simulink model "power_PSTdeltahex"  (Simulink 6.0)
settings: Solver=ode23tb  StartTime=0.0  StopTime=50  MaxStep=1/60  RelTol=1e-4  AbsTol=1e-3
undefined symbols (not defined in the file or in its folder): I21_init_imag, I21_init_real
libraries: powerlib x117, powerlib_extras x19, simulink_extras x1
(part 3 of 3)

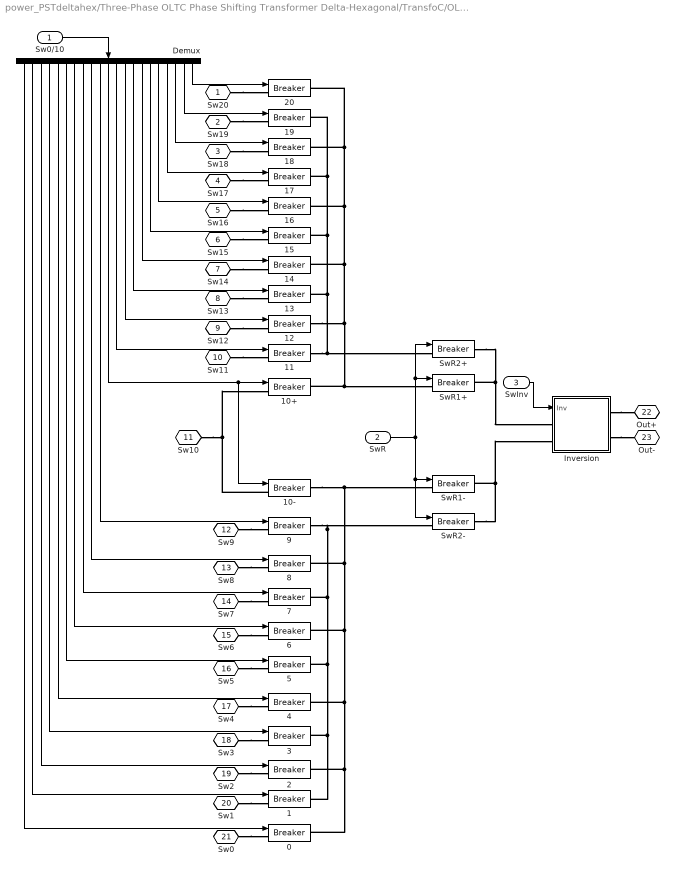
== system power_PSTdeltahex/Three-Phase OLTC Phase Shifting Transformer Delta-Hexagonal/TransfoC/OLTC ==
  Sw0/10 : Inport  Port=1  LatchInput=off
  SwR : Inport  Port=2  LatchInput=off
  SwInv : Inport  Port=3  LatchInput=off
  "0  " : powerlib/Elements/Breaker  BreakerResistance=Ron  InitialState=InitialStates(1)  SnubberResistance=Rsnub  SnubberCapacitance=inf  SwitchingTimes="[ 1/60  5/60 ]"  External=on  Measurements=None
  "1  " : powerlib/Elements/Breaker  BreakerResistance=Ron  InitialState=InitialStates(2)  SnubberResistance=Rsnub  SnubberCapacitance=inf  SwitchingTimes="[ 1/60  5/60 ]"  External=on  Measurements=None
  "10+  " : powerlib/Elements/Breaker  BreakerResistance=Ron  InitialState=InitialStates(11)  SnubberResistance=1e6  SnubberCapacitance=Rsnub  SwitchingTimes="[ 1/60  5/60 ]"  External=on  Measurements=None
  10- : powerlib/Elements/Breaker  BreakerResistance=Ron  InitialState=InitialStates(11)  SnubberResistance=Rsnub  SnubberCapacitance=inf  SwitchingTimes="[ 1/60  5/60 ]"  External=on  Measurements=None
  11 : powerlib/Elements/Breaker  BreakerResistance=Ron  InitialState=InitialStates(12)  SnubberResistance=Rsnub  SnubberCapacitance=inf  SwitchingTimes="[ 1/60  5/60 ]"  External=on  Measurements=None
  12 : powerlib/Elements/Breaker  BreakerResistance=Ron  InitialState=InitialStates(13)  SnubberResistance=Rsnub  SnubberCapacitance=inf  SwitchingTimes="[ 1/60  5/60 ]"  External=on  Measurements=None
  13 : powerlib/Elements/Breaker  BreakerResistance=Ron  InitialState=InitialStates(14)  SnubberResistance=Rsnub  SnubberCapacitance=inf  SwitchingTimes="[ 1/60  5/60 ]"  External=on  Measurements=None
  14 : powerlib/Elements/Breaker  BreakerResistance=Ron  InitialState=InitialStates(15)  SnubberResistance=Rsnub  SnubberCapacitance=inf  SwitchingTimes="[ 1/60  5/60 ]"  External=on  Measurements=None
  15 : powerlib/Elements/Breaker  BreakerResistance=Ron  InitialState=InitialStates(16)  SnubberResistance=Rsnub  SnubberCapacitance=inf  SwitchingTimes="[ 1/60  5/60 ]"  External=on  Measurements=None
  "16  " : powerlib/Elements/Breaker  BreakerResistance=Ron  InitialState=InitialStates(17)  SnubberResistance=Rsnub  SnubberCapacitance=inf  SwitchingTimes="[ 1/60  5/60 ]"  External=on  Measurements=None
  17 : powerlib/Elements/Breaker  BreakerResistance=Ron  InitialState=InitialStates(18)  SnubberResistance=Rsnub  SnubberCapacitance=inf  SwitchingTimes="[ 1/60  5/60 ]"  External=on  Measurements=None
  18 : powerlib/Elements/Breaker  BreakerResistance=Ron  InitialState=InitialStates(19)  SnubberResistance=Rsnub  SnubberCapacitance=inf  SwitchingTimes="[ 1/60  5/60 ]"  External=on  Measurements=None
  19 : powerlib/Elements/Breaker  BreakerResistance=Ron  InitialState=InitialStates(20)  SnubberResistance=Rsnub  SnubberCapacitance=inf  SwitchingTimes="[ 1/60  5/60 ]"  External=on  Measurements=None
  "2    " : powerlib/Elements/Breaker  BreakerResistance=Ron  InitialState=InitialStates(3)  SnubberResistance=Rsnub  SnubberCapacitance=inf  SwitchingTimes="[ 1/60  5/60 ]"  External=on  Measurements=None
  20 : powerlib/Elements/Breaker  BreakerResistance=Ron  InitialState=InitialStates(21)  SnubberResistance=Rsnub  SnubberCapacitance=inf  SwitchingTimes="[ 1/60  5/60 ]"  External=on  Measurements=None
  "3  " : powerlib/Elements/Breaker  BreakerResistance=Ron  InitialState=InitialStates(4)  SnubberResistance=Rsnub  SnubberCapacitance=inf  SwitchingTimes="[ 1/60  5/60 ]"  External=on  Measurements=None
  "4  " : powerlib/Elements/Breaker  BreakerResistance=Ron  InitialState=InitialStates(5)  SnubberResistance=Rsnub  SnubberCapacitance=inf  SwitchingTimes="[ 1/60  5/60 ]"  External=on  Measurements=None
  5 : powerlib/Elements/Breaker  BreakerResistance=Ron  InitialState=InitialStates(6)  SnubberResistance=Rsnub  SnubberCapacitance=inf  SwitchingTimes="[ 1/60  5/60 ]"  External=on  Measurements=None
  6 : powerlib/Elements/Breaker  BreakerResistance=Ron  InitialState=InitialStates(7)  SnubberResistance=Rsnub  SnubberCapacitance=inf  SwitchingTimes="[ 1/60  5/60 ]"  External=on  Measurements=None
  7 : powerlib/Elements/Breaker  BreakerResistance=Ron  InitialState=InitialStates(8)  SnubberResistance=Rsnub  SnubberCapacitance=inf  SwitchingTimes="[ 1/60  5/60 ]"  External=on  Measurements=None
  8 : powerlib/Elements/Breaker  BreakerResistance=Ron  InitialState=InitialStates(9)  SnubberResistance=Rsnub  SnubberCapacitance=inf  SwitchingTimes="[ 1/60  5/60 ]"  External=on  Measurements=None
  9 : powerlib/Elements/Breaker  BreakerResistance=Ron  InitialState=InitialStates(10)  SnubberResistance=Rsnub  SnubberCapacitance=inf  SwitchingTimes="[ 1/60  5/60 ]"  External=on  Measurements=None
  Demux : Demux  Orientation=down  Outputs=21
  Inversion : Subsystem
  SwR1+ : powerlib/Elements/Breaker  BreakerResistance=Ron  InitialState=1  SnubberResistance=R  SnubberCapacitance=inf  SwitchingTimes="[ 1/60  5/60 ]"  External=on  Measurements=None
  SwR1- : powerlib/Elements/Breaker  BreakerResistance=Ron  InitialState=1  SnubberResistance=R  SnubberCapacitance=inf  SwitchingTimes="[ 1/60  5/60 ]"  External=on  Measurements=None
  SwR2+ : powerlib/Elements/Breaker  BreakerResistance=Ron  InitialState=1  SnubberResistance=R  SnubberCapacitance=inf  SwitchingTimes="[ 1/60  5/60 ]"  External=on  Measurements=None
  SwR2- : powerlib/Elements/Breaker  BreakerResistance=Ron  InitialState=1  SnubberResistance=R  SnubberCapacitance=inf  SwitchingTimes="[ 1/60  5/60 ]"  External=on  Measurements=None
  Sw20 : PMIOPort  Port=1  Side=Left
  Sw19 : PMIOPort  Port=2  Side=Left
  Sw18 : PMIOPort  Port=3  Side=Left
  Sw17 : PMIOPort  Port=4  Side=Left
  Sw16 : PMIOPort  Port=5  Side=Left
  Sw15 : PMIOPort  Port=6  Side=Left
  Sw14 : PMIOPort  Port=7  Side=Left
  Sw13 : PMIOPort  Port=8  Side=Left
  Sw12 : PMIOPort  Port=9  Side=Left
  Sw11 : PMIOPort  Port=10  Side=Left
  Sw10 : PMIOPort  Port=11  Side=Left
  "Sw9 " : PMIOPort  Port=12  Side=Left
  Sw8 : PMIOPort  Port=13  Side=Left
  Sw7 : PMIOPort  Port=14  Side=Left
  Sw6 : PMIOPort  Port=15  Side=Left
  Sw5 : PMIOPort  Port=16  Side=Left
  Sw4 : PMIOPort  Port=17  Side=Left
  Sw3 : PMIOPort  Port=18  Side=Left
  "Sw2 " : PMIOPort  Port=19  Side=Left
  Sw1 : PMIOPort  Port=20  Side=Left
  Sw0 : PMIOPort  Port=21  Side=Left
  Out+ : PMIOPort  Orientation=left  Port=22  Side=Right
  Out- : PMIOPort  Orientation=left  Port=23  Side=Right
  wires:
  Sw0/10/1 -> Demux/1
  Demux/1 -> "0  "/1
  Demux/2 -> "1  "/1
  Demux/3 -> "2    "/1
  Demux/4 -> "3  "/1
  Demux/5 -> "4  "/1
  SwInv/1 -> Inversion/1(Inv)
  Demux/21 -> 20/1
  Demux/20 -> 19/1
  Demux/19 -> 18/1
  Demux/18 -> 17/1
  Demux/17 -> "16  "/1
  Demux/16 -> 15/1
  Demux/15 -> 14/1
  Demux/14 -> 13/1
  Demux/13 -> 12/1
  Demux/12 -> 11/1
  Demux/11 -> "10+  "/1, 10-/1
  Demux/10 -> 9/1
  Demux/9 -> 8/1
  Demux/8 -> 7/1
  Demux/7 -> 6/1
  Demux/6 -> 5/1
  SwR/1 -> SwR2+/1, SwR1+/1, SwR1-/1, SwR2-/1
  connections:
  Sw20/RConn1 -- 20/LConn1
  Sw19/RConn1 -- 19/LConn1
  Sw18/RConn1 -- 18/LConn1
  Sw17/RConn1 -- 17/LConn1
  Sw16/RConn1 -- "16  "/LConn1
  Sw4/RConn1 -- "4  "/LConn1
  Sw3/RConn1 -- "3  "/LConn1
  "Sw2 "/RConn1 -- "2    "/LConn1
  Sw1/RConn1 -- "1  "/LConn1
  Sw0/RConn1 -- "0  "/LConn1
  Inversion/RConn1 -- Out+/RConn1
  Inversion/RConn2 -- Out-/RConn1
  Sw5/RConn1 -- 5/LConn1
  Sw6/RConn1 -- 6/LConn1
  Sw7/RConn1 -- 7/LConn1
  Sw8/RConn1 -- 8/LConn1
  "Sw9 "/RConn1 -- 9/LConn1
  Sw15/RConn1 -- 15/LConn1
  Sw14/RConn1 -- 14/LConn1
  Sw13/RConn1 -- 13/LConn1
  Sw12/RConn1 -- 12/LConn1
  Sw11/RConn1 -- 11/LConn1
  SwR2-/RConn1 -- SwR1-/RConn1 -- Inversion/LConn2
  10-/RConn1 -- 8/RConn1 -- 6/RConn1 -- "4  "/RConn1 -- "2    "/RConn1 -- "0  "/RConn1 -- SwR1-/LConn1
  9/RConn1 -- 7/RConn1 -- 5/RConn1 -- "3  "/RConn1 -- "1  "/RConn1 -- SwR2-/LConn1
  12/RConn1 -- 14/RConn1 -- "16  "/RConn1 -- 18/RConn1 -- 20/RConn1 -- "10+  "/RConn1 -- SwR1+/LConn1
  11/RConn1 -- 13/RConn1 -- 15/RConn1 -- 17/RConn1 -- 19/RConn1 -- SwR2+/LConn1
  10-/LConn1 -- "10+  "/LConn1 -- Sw10/RConn1
  SwR2+/RConn1 -- SwR1+/RConn1 -- Inversion/LConn1

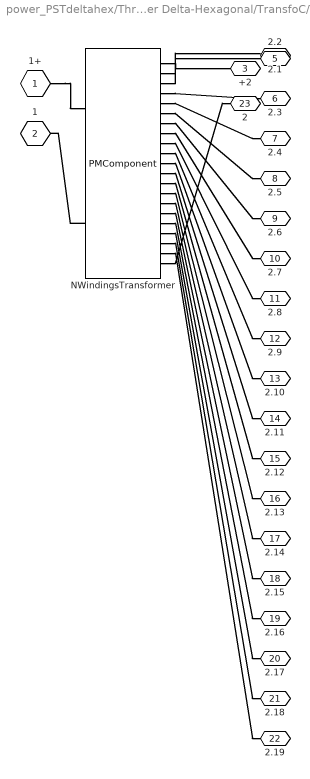
== system power_PSTdeltahex/Three-Phase OLTC Phase Shifting Transformer Delta-Hexagonal/TransfoC/Transformer ==
  NWindingsTransformer : PMComponent  PhysicalDomain=powersysdomain  LeftPortType=p1  RightPortType=p1  LConnTagsString=1|2  RConnTagsString=1|2|3|4|5|6|7|8|9|10|11|12|13|14|15|16|17|18|19|20|21
      mask Type: InnerPowersysBlock
  1+ : PMIOPort  Port=1  Side=Left
  1 : PMIOPort  Port=2  Side=Left
  +2 : PMIOPort  Orientation=left  Port=3  Side=Right
  2.1 : PMIOPort  Orientation=left  Port=4  Side=Right
  2.2 : PMIOPort  Orientation=left  Port=5  Side=Right
  2.3 : PMIOPort  Orientation=left  Port=6  Side=Right
  2.4 : PMIOPort  Orientation=left  Port=7  Side=Right
  2.5 : PMIOPort  Orientation=left  Port=8  Side=Right
  2.6 : PMIOPort  Orientation=left  Port=9  Side=Right
  2.7 : PMIOPort  Orientation=left  Port=10  Side=Right
  2.8 : PMIOPort  Orientation=left  Port=11  Side=Right
  2.9 : PMIOPort  Orientation=left  Port=12  Side=Right
  2.10 : PMIOPort  Orientation=left  Port=13  Side=Right
  2.11 : PMIOPort  Orientation=left  Port=14  Side=Right
  2.12 : PMIOPort  Orientation=left  Port=15  Side=Right
  2.13 : PMIOPort  Orientation=left  Port=16  Side=Right
  2.14 : PMIOPort  Orientation=left  Port=17  Side=Right
  2.15 : PMIOPort  Orientation=left  Port=18  Side=Right
  2.16 : PMIOPort  Orientation=left  Port=19  Side=Right
  2.17 : PMIOPort  Orientation=left  Port=20  Side=Right
  2.18 : PMIOPort  Orientation=left  Port=21  Side=Right
  2.19 : PMIOPort  Orientation=left  Port=22  Side=Right
  2 : PMIOPort  Orientation=left  Port=23  Side=Right
  connections:
  NWindingsTransformer/RConn1 -- +2/RConn1
  1+/RConn1 -- NWindingsTransformer/LConn1
  NWindingsTransformer/LConn2 -- 1/RConn1
  NWindingsTransformer/RConn2 -- 2.1/RConn1
  NWindingsTransformer/RConn3 -- 2.2/RConn1
  NWindingsTransformer/RConn4 -- 2.3/RConn1
  NWindingsTransformer/RConn5 -- 2.4/RConn1
  NWindingsTransformer/RConn6 -- 2.5/RConn1
  NWindingsTransformer/RConn7 -- 2.6/RConn1
  NWindingsTransformer/RConn8 -- 2.7/RConn1
  NWindingsTransformer/RConn9 -- 2.8/RConn1
  NWindingsTransformer/RConn10 -- 2.9/RConn1
  NWindingsTransformer/RConn21 -- 2/RConn1
  NWindingsTransformer/RConn11 -- 2.10/RConn1
  NWindingsTransformer/RConn12 -- 2.11/RConn1
  NWindingsTransformer/RConn13 -- 2.12/RConn1
  NWindingsTransformer/RConn14 -- 2.13/RConn1
  NWindingsTransformer/RConn15 -- 2.14/RConn1
  NWindingsTransformer/RConn16 -- 2.15/RConn1
  NWindingsTransformer/RConn17 -- 2.16/RConn1
  NWindingsTransformer/RConn18 -- 2.17/RConn1
  NWindingsTransformer/RConn19 -- 2.18/RConn1
  NWindingsTransformer/RConn20 -- 2.19/RConn1

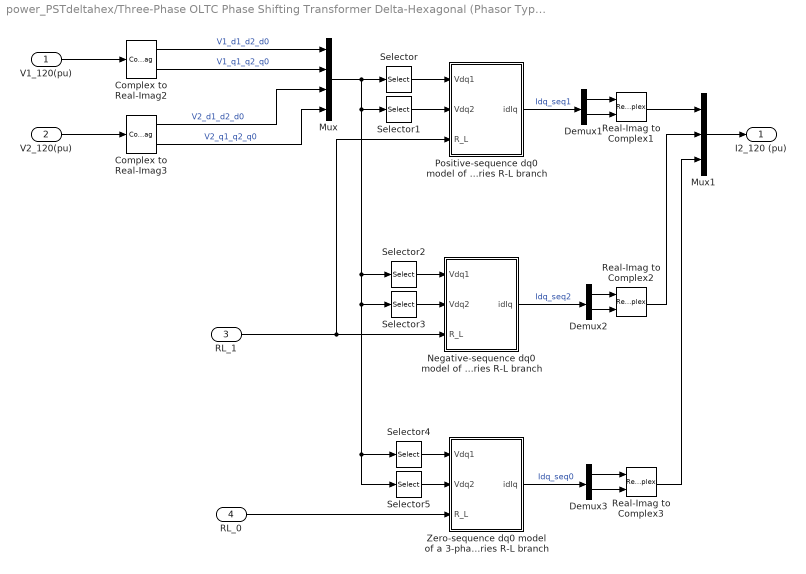
== system power_PSTdeltahex/Three-Phase OLTC Phase Shifting Transformer Delta-Hexagonal (Phasor Type)/ Currents/dq0 model of 3-ph RL branch ==
  V1_120(pu) : Inport  Port=1  LatchInput=off
  V2_120(pu) : Inport  Port=2  LatchInput=off
  RL_1 : Inport  Port=3  LatchInput=off
  RL_0 : Inport  Port=4  LatchInput=off
  Complex to Real-Imag2 : ComplexToRealImag
  Complex to Real-Imag3 : ComplexToRealImag
  Demux1 : Demux  Outputs=2
  Demux2 : Demux  Outputs=2
  Demux3 : Demux  Outputs=2
  Mux : Mux
  Mux1 : Mux  Inputs=3
  Negative-sequence dq0 model of a 3-phase series R-L branch : Subsystem
  Positive-sequence dq0 model of a 3-phase series R-L branch : Subsystem
  Real-Imag to Complex1 : RealImagToComplex
  Real-Imag to Complex2 : RealImagToComplex
  Real-Imag to Complex3 : RealImagToComplex
  Selector : Selector  Elements=[1 4]  InputPortWidth=12
  Selector1 : Selector  Elements=[7 10]  InputPortWidth=12
  Selector2 : Selector  Elements=[1 4]+1  InputPortWidth=12
  Selector3 : Selector  Elements=[7 10]+1  InputPortWidth=12
  Selector4 : Selector  Elements=[1 4]+2  InputPortWidth=12
  Selector5 : Selector  Elements=[7 10]+2  InputPortWidth=12
  Zero-sequence dq0 model of a 3-phase series R-L branch : Subsystem
  I2_120 (pu) : Outport
  wires:
  Positive-sequence dq0 model of a 3-phase series R-L branch/1(idIq) -> Demux1/1  "Idq_seq1"
  V1_120(pu)/1 -> Complex to Real-Imag2/1
  V2_120(pu)/1 -> Complex to Real-Imag3/1
  Selector/1 -> Positive-sequence dq0 model of a 3-phase series R-L branch/1(Vdq1)
  Selector1/1 -> Positive-sequence dq0 model of a 3-phase series R-L branch/2(Vdq2)
  Mux/1 -> Selector/1, Selector1/1, Selector2/1, Selector3/1, Selector4/1, Selector5/1
  Selector2/1 -> Negative-sequence dq0 model of a 3-phase series R-L branch/1(Vdq1)
  Selector3/1 -> Negative-sequence dq0 model of a 3-phase series R-L branch/2(Vdq2)
  Selector4/1 -> Zero-sequence dq0 model of a 3-phase series R-L branch/1(Vdq1)
  Negative-sequence dq0 model of a 3-phase series R-L branch/1(idIq) -> Demux2/1  "Idq_seq2"
  Zero-sequence dq0 model of a 3-phase series R-L branch/1(idIq) -> Demux3/1  "Idq_seq0"
  Complex to Real-Imag2/1 -> Mux/1  "V1_d1_d2_d0"
  Complex to Real-Imag2/2 -> Mux/2  "V1_q1_q2_q0"
  Complex to Real-Imag3/1 -> Mux/3  "V2_d1_d2_d0"
  Complex to Real-Imag3/2 -> Mux/4  "V2_q1_q2_q0"
  RL_1/1 -> Positive-sequence dq0 model of a 3-phase series R-L branch/3(R_L), Negative-sequence dq0 model of a 3-phase series R-L branch/3(R_L)
  Selector5/1 -> Zero-sequence dq0 model of a 3-phase series R-L branch/2(Vdq2)
  RL_0/1 -> Zero-sequence dq0 model of a 3-phase series R-L branch/3(R_L)
  Demux1/2 -> Real-Imag to Complex1/2
  Demux1/1 -> Real-Imag to Complex1/1
  Real-Imag to Complex1/1 -> Mux1/1
  Demux2/2 -> Real-Imag to Complex2/2
  Demux2/1 -> Real-Imag to Complex2/1
  Real-Imag to Complex2/1 -> Mux1/2
  Demux3/2 -> Real-Imag to Complex3/2
  Demux3/1 -> Real-Imag to Complex3/1
  Real-Imag to Complex3/1 -> Mux1/3
  Mux1/1 -> I2_120 (pu)/1

== system power_PSTdeltahex/Three-Phase OLTC Phase Shifting Transformer Delta-Hexagonal (Phasor Type)/Tap Changer Control/Determine tap positon ==
  NewTap : Inport  Port=1  LatchInput=off
  Trigger : TriggerPort
  Memory : Memory  Orientation=left  X0=InitialPosition  InheritSampleTime=on
  Saturation : Saturate  UpperLimit=MinMaxTap(2)  LowerLimit=MinMaxTap(1)
  Sum : Sum  Inputs=|++  SaturateOnIntegerOverflow=on
  TapNo : Outport  InitialOutput=InitialPosition
  wires:
  NewTap/1 -> Sum/1
  Sum/1 -> Saturation/1
  Memory/1 -> Sum/2
  Saturation/1 -> TapNo/1, Memory/1

== system power_PSTdeltahex/Three-Phase OLTC Phase Shifting Transformer Delta-Hexagonal/OLTC Control/Monostable/Edge Detector ==
  note: Silvano Casoria
      | Power System Simulation Laboratory
      | IREQ, Hydro-Quebec
  note: Edge or Slope Detector
  In : Inport  Port=1  LatchInput=off
  Constant1 : Constant  Value=model
  Demux : Demux  Outputs=2
  Logical Operator1 : Logic  Operator=OR
  Memory : Memory  X0=ic  InheritSampleTime=on
  Multiport Switch : MultiPortSwitch  Inputs=3  SaturateOnIntegerOverflow=on
  NEGATIVE Edge : Subsystem  AncestorBlock=extra_sc/Edge/POSITIVE Edge  TreatAsAtomicUnit=on
  POSITIVE Edge : Subsystem  AncestorBlock=extra_sc/Delay_discrete/OFF Delay  TreatAsAtomicUnit=on
  either edge : Constant  Value=[1 1]
  neg. edge : Constant  Value=[0 1]
  pos. edge : Constant  Value=[1 0]
  Out : Outport
  wires:
  Logical Operator1/1 -> Out/1
  NEGATIVE Edge/1(OUT) -> Logical Operator1/2
  POSITIVE Edge/1(OUT) -> Logical Operator1/1
  Memory/1 -> POSITIVE Edge/2(IN previous), NEGATIVE Edge/2(IN previous)
  In/1 -> POSITIVE Edge/1(IN), NEGATIVE Edge/1(IN), Memory/1
  pos. edge/1 -> Multiport Switch/2
  neg. edge/1 -> Multiport Switch/3
  Constant1/1 -> Multiport Switch/1
  Multiport Switch/1 -> Demux/1
  Demux/1 -> POSITIVE Edge/Enable
  Demux/2 -> NEGATIVE Edge/Enable
  either edge/1 -> Multiport Switch/4

== system power_PSTdeltahex/Three-Phase OLTC Phase Shifting Transformer Delta-Hexagonal/OLTC Control/Tap Changer Control/Determine tap positon ==
  NewTap : Inport  Port=1  LatchInput=off
  Trigger : TriggerPort
  Memory : Memory  Orientation=left  X0=InitialPosition  InheritSampleTime=on
  Saturation : Saturate  UpperLimit=MinMaxTap(2)  LowerLimit=MinMaxTap(1)
  Sum : Sum  Inputs=|++  SaturateOnIntegerOverflow=on
  TapNo : Outport  InitialOutput=InitialPosition
  wires:
  Saturation/1 -> Memory/1, TapNo/1
  Memory/1 -> Sum/2
  Sum/1 -> Saturation/1
  NewTap/1 -> Sum/1

== system power_PSTdeltahex/Three-Phase OLTC Phase Shifting Transformer Delta-Hexagonal/TransfoA/OLTC/Inversion ==
  Inv : Inport  Port=1  LatchInput=off
  Logical Operator : Logic  Operator=NOT  AllPortsSameDT=off
  SwInv1 : powerlib/Elements/Breaker  BreakerResistance=Ron  InitialState=1  SnubberResistance=Rsnub  SnubberCapacitance=inf  SwitchingTimes="[ 1/60  5/60 ]"  External=on  Measurements=None
  SwInv2 : powerlib/Elements/Breaker  BreakerResistance=Ron  InitialState=0  SnubberResistance=Rsnub  SnubberCapacitance=inf  SwitchingTimes="[ 1/60  5/60 ]"  External=on  Measurements=None
  SwInv3 : powerlib/Elements/Breaker  BreakerResistance=Ron  InitialState=1  SnubberResistance=Rsnub  SnubberCapacitance=inf  SwitchingTimes="[ 1/60  5/60 ]"  External=on  Measurements=None
  SwInv4 : powerlib/Elements/Breaker  BreakerResistance=Ron  InitialState=0  SnubberResistance=Rsnub  SnubberCapacitance=inf  SwitchingTimes="[ 1/60  5/60 ]"  External=on  Measurements=None
  In1 : PMIOPort  Port=1  Side=Left
  In2 : PMIOPort  Port=2  Side=Left
  Out1 : PMIOPort  Orientation=left  Port=3  Side=Right
  Out2 : PMIOPort  Orientation=left  Port=4  Side=Right
  wires:
  Inv/1 -> SwInv1/1, SwInv3/1, Logical Operator/1
  Logical Operator/1 -> SwInv2/1, SwInv4/1
  connections:
  SwInv1/RConn1 -- SwInv4/RConn1 -- Out1/RConn1
  In1/RConn1 -- SwInv1/LConn1 -- SwInv2/LConn1
  SwInv3/RConn1 -- SwInv2/RConn1 -- Out2/RConn1
  In2/RConn1 -- SwInv3/LConn1 -- SwInv4/LConn1

== system power_PSTdeltahex/Three-Phase OLTC Phase Shifting Transformer Delta-Hexagonal/TransfoB/OLTC/Inversion ==
  Inv : Inport  Port=1  LatchInput=off
  Logical Operator : Logic  Operator=NOT  AllPortsSameDT=off
  SwInv1 : powerlib/Elements/Breaker  BreakerResistance=Ron  InitialState=1  SnubberResistance=Rsnub  SnubberCapacitance=inf  SwitchingTimes="[ 1/60  5/60 ]"  External=on  Measurements=None
  SwInv2 : powerlib/Elements/Breaker  BreakerResistance=Ron  InitialState=0  SnubberResistance=Rsnub  SnubberCapacitance=inf  SwitchingTimes="[ 1/60  5/60 ]"  External=on  Measurements=None
  SwInv3 : powerlib/Elements/Breaker  BreakerResistance=Ron  InitialState=1  SnubberResistance=Rsnub  SnubberCapacitance=inf  SwitchingTimes="[ 1/60  5/60 ]"  External=on  Measurements=None
  SwInv4 : powerlib/Elements/Breaker  BreakerResistance=Ron  InitialState=0  SnubberResistance=Rsnub  SnubberCapacitance=inf  SwitchingTimes="[ 1/60  5/60 ]"  External=on  Measurements=None
  In1 : PMIOPort  Port=1  Side=Left
  In2 : PMIOPort  Port=2  Side=Left
  Out1 : PMIOPort  Orientation=left  Port=3  Side=Right
  Out2 : PMIOPort  Orientation=left  Port=4  Side=Right
  wires:
  Logical Operator/1 -> SwInv4/1, SwInv2/1
  Inv/1 -> Logical Operator/1, SwInv3/1, SwInv1/1
  connections:
  SwInv4/LConn1 -- SwInv3/LConn1 -- In2/RConn1
  Out2/RConn1 -- SwInv2/RConn1 -- SwInv3/RConn1
  SwInv2/LConn1 -- SwInv1/LConn1 -- In1/RConn1
  Out1/RConn1 -- SwInv4/RConn1 -- SwInv1/RConn1

== system power_PSTdeltahex/Three-Phase OLTC Phase Shifting Transformer Delta-Hexagonal/TransfoC/OLTC/Inversion ==
  Inv : Inport  Port=1  LatchInput=off
  Logical Operator : Logic  Operator=NOT  AllPortsSameDT=off
  SwInv1 : powerlib/Elements/Breaker  BreakerResistance=Ron  InitialState=1  SnubberResistance=Rsnub  SnubberCapacitance=inf  SwitchingTimes="[ 1/60  5/60 ]"  External=on  Measurements=None
  SwInv2 : powerlib/Elements/Breaker  BreakerResistance=Ron  InitialState=0  SnubberResistance=Rsnub  SnubberCapacitance=inf  SwitchingTimes="[ 1/60  5/60 ]"  External=on  Measurements=None
  SwInv3 : powerlib/Elements/Breaker  BreakerResistance=Ron  InitialState=1  SnubberResistance=Rsnub  SnubberCapacitance=inf  SwitchingTimes="[ 1/60  5/60 ]"  External=on  Measurements=None
  SwInv4 : powerlib/Elements/Breaker  BreakerResistance=Ron  InitialState=0  SnubberResistance=Rsnub  SnubberCapacitance=inf  SwitchingTimes="[ 1/60  5/60 ]"  External=on  Measurements=None
  In1 : PMIOPort  Port=1  Side=Left
  In2 : PMIOPort  Port=2  Side=Left
  Out1 : PMIOPort  Orientation=left  Port=3  Side=Right
  Out2 : PMIOPort  Orientation=left  Port=4  Side=Right
  wires:
  Inv/1 -> SwInv1/1, SwInv3/1, Logical Operator/1
  Logical Operator/1 -> SwInv2/1, SwInv4/1
  connections:
  SwInv1/RConn1 -- SwInv4/RConn1 -- Out1/RConn1
  In1/RConn1 -- SwInv1/LConn1 -- SwInv2/LConn1
  SwInv3/RConn1 -- SwInv2/RConn1 -- Out2/RConn1
  In2/RConn1 -- SwInv3/LConn1 -- SwInv4/LConn1

== system power_PSTdeltahex/Three-Phase OLTC Phase Shifting Transformer Delta-Hexagonal (Phasor Type)/ Currents/dq0 model of 3-ph RL branch/Negative-sequence dq0 model of a 3-phase series R-L branch ==
  note: where w = 2*pi*Fnom (Hz)
  note: Vq1 - Vq2 = [ R * Iq ] + [ L* w * Id ] + [ L * d/dt (Iq) ]
  note: ==========================================================================================
  note: I --->
  note: V2
  note: V1
  note: o--------| R |---| L |-------o
  note: Vd1 - Vd2 = [ R * Id ] - [ L* w * Iq ] + [ L * d/dt (Id) ]
  note: where w = 2*pi*Fnom (Hz)
  note: Iq = [ w / ( L * s ) ] * [ Vq1 - Vq2 - ( R * Iq ) - ( L * Id ) ]
  note: Id = [ w / ( L * s ) ] * [ Vd1 - Vd2 - ( R * Id ) + ( L * Iq ) ]
  note: d-q axis model of a 3-phase series R-L branch
  note: Using Laplace transform and per unit (pu) quantities :
  Vdq1 : Inport  Port=1  LatchInput=off
  Vdq2 : Inport  Port=2  LatchInput=off
  R_L : Inport  Port=3  LatchInput=off
  Demux3 : Demux  Outputs=2
  Integrator : Integrator
  Product : Product  SaturateOnIntegerOverflow=on
  Product1 : Product  SaturateOnIntegerOverflow=on
  Product2 : Product  Inputs=*/  SaturateOnIntegerOverflow=on
  R_choke2 : Gain  Gain=[1 -1]  SaturateOnIntegerOverflow=on
  R_choke3 : Gain  Gain=w  SaturateOnIntegerOverflow=on
  Selector : Selector  Elements=[2 1]  InputPortWidth=2
  Sum : Sum  Inputs=+--+  SaturateOnIntegerOverflow=on
  idIq : Outport
  wires:
  Demux3/1 -> Product/2
  Demux3/2 -> Product1/2, Product2/2
  R_L/1 -> Demux3/1
  Product2/1 -> Integrator/1
  R_choke3/1 -> Product2/1
  Selector/1 -> Product1/1
  Integrator/1 -> Product/1, Selector/1, idIq/1
  Sum/1 -> R_choke3/1
  Product1/1 -> R_choke2/1
  R_choke2/1 -> Sum/4
  Product/1 -> Sum/3
  Vdq2/1 -> Sum/2
  Vdq1/1 -> Sum/1

== system power_PSTdeltahex/Three-Phase OLTC Phase Shifting Transformer Delta-Hexagonal (Phasor Type)/ Currents/dq0 model of 3-ph RL branch/Positive-sequence dq0 model of a 3-phase series R-L branch ==
  note: Using Laplace transform and per unit (pu) quantities :
  note: d-q axis model of a 3-phase series R-L branch
  note: Id = [ w / ( L * s ) ] * [ Vd1 - Vd2 - ( R * Id ) + ( L * Iq ) ]
  note: Iq = [ w / ( L * s ) ] * [ Vq1 - Vq2 - ( R * Iq ) - ( L * Id ) ]
  note: where w = 2*pi*Fnom (Hz)
  note: Vd1 - Vd2 = [ R * Id ] - [ L* w * Iq ] + [ L * d/dt (Id) ]
  note: o--------| R |---| L |-------o
  note: V1
  note: V2
  note: I --->
  note: ==========================================================================================
  note: Vq1 - Vq2 = [ R * Iq ] + [ L* w * Id ] + [ L * d/dt (Iq) ]
  note: where w = 2*pi*Fnom (Hz)
  Vdq1 : Inport  Port=1  LatchInput=off
  Vdq2 : Inport  Port=2  LatchInput=off
  R_L : Inport  Port=3  LatchInput=off
  Demux3 : Demux  Outputs=2
  Integrator : Integrator  InitialCondition="[I21_init_real   I21_init_imag]"
  Product : Product  SaturateOnIntegerOverflow=on
  Product1 : Product  SaturateOnIntegerOverflow=on
  Product2 : Product  Inputs=*/  SaturateOnIntegerOverflow=on
  R_choke2 : Gain  Gain=[1 -1]  SaturateOnIntegerOverflow=on
  R_choke3 : Gain  Gain=w  SaturateOnIntegerOverflow=on
  Selector : Selector  Elements=[2 1]  InputPortWidth=2
  Sum : Sum  Inputs=+--+  SaturateOnIntegerOverflow=on
  idIq : Outport
  wires:
  Vdq1/1 -> Sum/1
  Vdq2/1 -> Sum/2
  Product/1 -> Sum/3
  R_choke2/1 -> Sum/4
  Product1/1 -> R_choke2/1
  Sum/1 -> R_choke3/1
  Integrator/1 -> idIq/1, Selector/1, Product/1
  Selector/1 -> Product1/1
  R_choke3/1 -> Product2/1
  Product2/1 -> Integrator/1
  R_L/1 -> Demux3/1
  Demux3/2 -> Product2/2, Product1/2
  Demux3/1 -> Product/2

== system power_PSTdeltahex/Three-Phase OLTC Phase Shifting Transformer Delta-Hexagonal (Phasor Type)/ Currents/dq0 model of 3-ph RL branch/Zero-sequence dq0 model of a 3-phase series R-L branch ==
  note: Using Laplace transform and per unit (pu) quantities :
  note: d-q axis model of a 3-phase series R-L branch
  note: Id = [ w / ( L * s ) ] * [ Vd1 - Vd2 - ( R * Id ) + ( L * Iq ) ]
  note: Iq = [ w / ( L * s ) ] * [ Vq1 - Vq2 - ( R * Iq ) - ( L * Id ) ]
  note: where w = 2*pi*Fnom (Hz)
  note: Vd1 - Vd2 = [ R * Id ] - [ L* w * Iq ] + [ L * d/dt (Id) ]
  note: o--------| R |---| L |-------o
  note: V1
  note: V2
  note: I --->
  note: ==========================================================================================
  note: Vq1 - Vq2 = [ R * Iq ] + [ L* w * Id ] + [ L * d/dt (Iq) ]
  note: where w = 2*pi*Fnom (Hz)
  Vdq1 : Inport  Port=1  LatchInput=off
  Vdq2 : Inport  Port=2  LatchInput=off
  R_L : Inport  Port=3  LatchInput=off
  Demux3 : Demux  Outputs=2
  Integrator : Integrator
  Product : Product  SaturateOnIntegerOverflow=on
  Product1 : Product  SaturateOnIntegerOverflow=on
  Product2 : Product  Inputs=*/  SaturateOnIntegerOverflow=on
  R_choke2 : Gain  Gain=[1 -1]  SaturateOnIntegerOverflow=on
  R_choke3 : Gain  Gain=w  SaturateOnIntegerOverflow=on
  Selector : Selector  Elements=[2 1]  InputPortWidth=2
  Sum : Sum  Inputs=+--+  SaturateOnIntegerOverflow=on
  idIq : Outport
  wires:
  Vdq1/1 -> Sum/1
  Vdq2/1 -> Sum/2
  Product/1 -> Sum/3
  R_choke2/1 -> Sum/4
  Product1/1 -> R_choke2/1
  Sum/1 -> R_choke3/1
  Integrator/1 -> idIq/1, Selector/1, Product/1
  Selector/1 -> Product1/1
  R_choke3/1 -> Product2/1
  Product2/1 -> Integrator/1
  R_L/1 -> Demux3/1
  Demux3/2 -> Product2/2, Product1/2
  Demux3/1 -> Product/2

== system power_PSTdeltahex/Three-Phase OLTC Phase Shifting Transformer Delta-Hexagonal/OLTC Control/Monostable/Edge Detector/NEGATIVE Edge ==
  IN : Inport  Port=1  LatchInput=off
  IN previous : Inport  Port=2  LatchInput=off
  Enable : EnablePort
  Relational Operator1 : RelationalOperator  Operator=>  InputSameDT=on
  OUT : Outport
  wires:
  Relational Operator1/1 -> OUT/1
  IN previous/1 -> Relational Operator1/1
  IN/1 -> Relational Operator1/2

== system power_PSTdeltahex/Three-Phase OLTC Phase Shifting Transformer Delta-Hexagonal/OLTC Control/Monostable/Edge Detector/POSITIVE Edge ==
  IN : Inport  Port=1  LatchInput=off
  IN previous : Inport  Port=2  LatchInput=off
  Enable : EnablePort
  Relational Operator1 : RelationalOperator  Operator=>  InputSameDT=on
  OUT : Outport
  wires:
  Relational Operator1/1 -> OUT/1
  IN previous/1 -> Relational Operator1/2
  IN/1 -> Relational Operator1/1
